simulink model "Robot"  (R2019b)
settings: Solver=VariableStepAuto  StartTime=0.0  StopTime=20  RelTol=1e-3
undefined symbols (not defined in the file or in its folder): X, Y, Z
libraries: sm_lib x11, nesl_utility x7
settings Model: Creator=Usuario  LastModifiedBy=Usuario

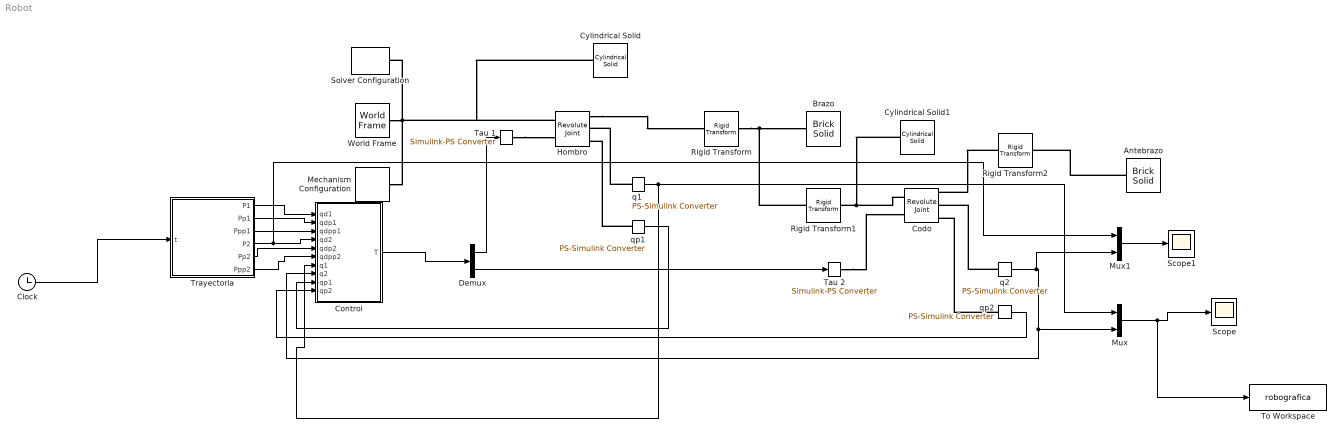
== system Robot ==
  " Brazo" : sm_lib/Body Elements/Brick Solid  GraphicAmbientColor=[0.15 0.15 0.15 1.0]  BasedOnType=Density  BrickDimensions=[0.1 1 0.1]  BrickDimensionUnits=m  CenterOfMass=[0 0 0]  CenterOfMassUnits=m  GraphicDiffuseColor=[1.0 0.2 0.2]  Density=1000  DensityUnits=kg/m^3  DoExposeReferenceFrame=on  GraphicEmissiveColor=[0.0 0.0 0.0 1.0]  ExportEntireGeometry=off  SerializedFrames=<Frames/>  MarkerShape=Sphere  MarkerSize=10  GraphicType=FromGeometry  InertiaType=Custom  Mass=1  MassUnits=kg  MomentsOfInertia=[1 1 0.01]  MomentsOfInertiaUnits=kg*m^2  GraphicOpacity=1.0  ProductsOfInertia=[0 0 0]  ProductsOfInertiaUnits=kg*m^2  GraphicShininess=75  GraphicSpecularColor=[0.5 0.5 0.5 1.0]  GraphicVisPropType=SimpleVisualProperties
  Antebrazo : sm_lib/Body Elements/Brick Solid  GraphicAmbientColor=[0.15 0.15 0.15 1.0]  BasedOnType=Density  BrickDimensions=[0.1 1 0.1]  BrickDimensionUnits=m  CenterOfMass=[0 0 0]  CenterOfMassUnits=m  GraphicDiffuseColor=[0.0 0.0 1.0]  Density=1000  DensityUnits=kg/m^3  DoExposeReferenceFrame=on  GraphicEmissiveColor=[0.0 0.0 0.0 1.0]  ExportEntireGeometry=off  SerializedFrames=<Frames/>  MarkerShape=Sphere  MarkerSize=10  GraphicType=FromGeometry  InertiaType=Custom  Mass=1  MassUnits=kg  MomentsOfInertia=[1 1 0.01]  MomentsOfInertiaUnits=kg*m^2  GraphicOpacity=1.0  ProductsOfInertia=[0 0 0]  ProductsOfInertiaUnits=kg*m^2  GraphicShininess=75  GraphicSpecularColor=[0.5 0.5 0.5 1.0]  GraphicVisPropType=SimpleVisualProperties
  Clock : Clock
  Codo : sm_lib/Joints/Revolute Joint  JointMode=Normal  SenseConstraintForce=off  SenseConstraintForceX=off  SenseConstraintForceY=off  SenseConstraintForceZ=off  SenseConstraintTorque=off  SenseConstraintTorqueX=off  SenseConstraintTorqueY=off  SenseConstraintTorqueZ=off  SenseTotalForce=off  SenseTotalForceX=off  SenseTotalForceY=off  SenseTotalForceZ=off  SenseTotalTorque=off  SenseTotalTorqueX=off  SenseTotalTorqueY=off  SenseTotalTorqueZ=off  CompositeWrenchDir=FollowerOnBase  CompositeWrenchFrame=BaseFrame  EquilibriumPosition=0  EquilibriumPositionUnits=deg  SpringStiffness=0  SpringStiffnessUnits=N*m/deg  DampingCoefficient=0.13  DampingCoefficientUnits=N*m/(rad/s)  TorqueActuationMode=InputTorque  MotionActuationMode=ComputedMotion  SensePosition=on  SenseVelocity=on  SenseAcceleration=off  SenseTorqueForce=off  SenseLowerLimitTorqueForce=off  SenseUpperLimitTorqueForce=off  LowerLimitSpecify=off  LowerLimitBound=-90  LowerLimitBoundUnits=deg  LowerLimitStiffness=1e4  LowerLimitStiffnessUnits=N*m/deg  LowerLimitDamping=10  LowerLimitDampingUnits=N*m/(deg/s)  LowerLimitTransitionRegionWidth=0.1  LowerLimitTransitionRegionWidthUnits=deg  UpperLimitSpecify=off  UpperLimitBound=90  UpperLimitBoundUnits=deg  UpperLimitStiffness=1e4  UpperLimitStiffnessUnits=N*m/deg  UpperLimitDamping=10  UpperLimitDampingUnits=N*m/(deg/s)  UpperLimitTransitionRegionWidth=0.1  UpperLimitTransitionRegionWidthUnits=deg  PositionTargetSpecify=on  PositionTargetPriority=High  PositionTargetValue=-pi/2  PositionTargetValueUnits=rad  VelocityTargetSpecify=off  VelocityTargetPriority=High  VelocityTargetValue=0  VelocityTargetValueUnits=deg/s
  Control : MATLAB Function  TreatAsAtomicUnit=on
  Cylindrical Solid : sm_lib/Body Elements/Cylindrical Solid  GraphicAmbientColor=[0.15 0.15 0.15 1.0]  BasedOnType=Density  CenterOfMass=[0 0 0]  CenterOfMassUnits=m  GraphicDiffuseColor=[1.0 1.0 0.0]  CylinderLength=0.12  CylinderLengthUnits=m  CylinderRadius=0.05  CylinderRadiusUnits=m  Density=1000  DensityUnits=kg/m^3  DoExposeReferenceFrame=on  GraphicEmissiveColor=[0.0 0.0 0.0 1.0]  ExportEntireGeometry=off  SerializedFrames=<Frames/>  MarkerShape=Sphere  MarkerSize=10  GraphicType=FromGeometry  InertiaType=Custom  Mass=0.0001  MassUnits=kg  MomentsOfInertia=[1 1 0.001]  MomentsOfInertiaUnits=kg*m^2  GraphicOpacity=1.0  ProductsOfInertia=[0 0 0]  ProductsOfInertiaUnits=kg*m^2  GraphicShininess=75  GraphicSpecularColor=[0.5 0.5 0.5 1.0]  GraphicVisPropType=SimpleVisualProperties
  Cylindrical Solid1 : sm_lib/Body Elements/Cylindrical Solid  GraphicAmbientColor=[0.15 0.15 0.15 1.0]  BasedOnType=Density  CenterOfMass=[0 0 0]  CenterOfMassUnits=m  GraphicDiffuseColor=[1.0 1.0 0.0]  CylinderLength=0.12  CylinderLengthUnits=m  CylinderRadius=0.05  CylinderRadiusUnits=m  Density=1000  DensityUnits=kg/m^3  DoExposeReferenceFrame=on  GraphicEmissiveColor=[0.0 0.0 0.0 1.0]  ExportEntireGeometry=off  SerializedFrames=<Frames/>  MarkerShape=Sphere  MarkerSize=10  GraphicType=FromGeometry  InertiaType=Custom  Mass=0.0001  MassUnits=kg  MomentsOfInertia=[1 1 0.001]  MomentsOfInertiaUnits=kg*m^2  GraphicOpacity=1.0  ProductsOfInertia=[0 0 0]  ProductsOfInertiaUnits=kg*m^2  GraphicShininess=75  GraphicSpecularColor=[0.5 0.5 0.5 1.0]  GraphicVisPropType=SimpleVisualProperties
  Demux : Demux  Outputs=2
  Hombro : sm_lib/Joints/Revolute Joint  JointMode=Normal  SenseConstraintForce=off  SenseConstraintForceX=off  SenseConstraintForceY=off  SenseConstraintForceZ=off  SenseConstraintTorque=off  SenseConstraintTorqueX=off  SenseConstraintTorqueY=off  SenseConstraintTorqueZ=off  SenseTotalForce=off  SenseTotalForceX=off  SenseTotalForceY=off  SenseTotalForceZ=off  SenseTotalTorque=off  SenseTotalTorqueX=off  SenseTotalTorqueY=off  SenseTotalTorqueZ=off  CompositeWrenchDir=FollowerOnBase  CompositeWrenchFrame=BaseFrame  EquilibriumPosition=0  EquilibriumPositionUnits=deg  SpringStiffness=0  SpringStiffnessUnits=N*m/deg  DampingCoefficient=0.17  DampingCoefficientUnits=N*m/(rad/s)  TorqueActuationMode=InputTorque  MotionActuationMode=ComputedMotion  SensePosition=on  SenseVelocity=on  SenseAcceleration=off  SenseTorqueForce=off  SenseLowerLimitTorqueForce=off  SenseUpperLimitTorqueForce=off  LowerLimitSpecify=off  LowerLimitBound=-90  LowerLimitBoundUnits=deg  LowerLimitStiffness=1e4  LowerLimitStiffnessUnits=N*m/deg  LowerLimitDamping=10  LowerLimitDampingUnits=N*m/(deg/s)  LowerLimitTransitionRegionWidth=0.1  LowerLimitTransitionRegionWidthUnits=deg  UpperLimitSpecify=off  UpperLimitBound=90  UpperLimitBoundUnits=deg  UpperLimitStiffness=1e4  UpperLimitStiffnessUnits=N*m/deg  UpperLimitDamping=10  UpperLimitDampingUnits=N*m/(deg/s)  UpperLimitTransitionRegionWidth=0.1  UpperLimitTransitionRegionWidthUnits=deg  PositionTargetSpecify=off  PositionTargetPriority=High  PositionTargetValue=pi/2  PositionTargetValueUnits=rad  VelocityTargetSpecify=off  VelocityTargetPriority=High  VelocityTargetValue=0  VelocityTargetValueUnits=deg/s
  Mechanism Configuration : sm_lib/Utilities/Mechanism Configuration  UniformGravity=Constant  GravityVector=[0 -9.80665 0]  GravityUnits=m/s^2  LinearizationDelta=0.001
  Mux : Mux  Inputs=2
  Mux1 : Mux  Inputs=2
  Rigid Transform : sm_lib/Frames and Transforms/Rigid Transform  TranslationMethod=Cartesian  TranslationStandardOffset=0  TranslationLengthUnit=m  TranslationStandardAxis=+Z  TranslationCartesianOffset=[0 -0.5 0]  TranslationROffset=0  TranslationROffsetUnits=m  TranslationZOffset=0  TranslationZOffsetUnits=m  TranslationThetaOffset=0  TranslationThetaOffsetUnits=deg  RotationMethod=None  RotationAngleUnits=deg  RotationStandardAxis=+Z  RotationAngle=0.0  RotationArbitraryAxis=[0 0 1]  FollAlignAxisA=+X  BaseAlignAxisA=+Y  FollAlignAxisB=+Y  BaseAlignAxisB=+Z  RotationSequenceAxes=FollowerAxes  RotationSequence=XYX  RotationSequenceAngles=[0 0 0]  RotationSequenceAnglesUnits=deg  RotationMatrix=[1 0 0; 0 1 0; 0 0 1]
  Rigid Transform1 : sm_lib/Frames and Transforms/Rigid Transform  TranslationMethod=Cartesian  TranslationStandardOffset=0  TranslationLengthUnit=m  TranslationStandardAxis=+Z  TranslationCartesianOffset=[0 -0.5 0]  TranslationROffset=0  TranslationROffsetUnits=m  TranslationZOffset=0  TranslationZOffsetUnits=m  TranslationThetaOffset=0  TranslationThetaOffsetUnits=deg  RotationMethod=None  RotationAngleUnits=deg  RotationStandardAxis=+Z  RotationAngle=0.0  RotationArbitraryAxis=[0 0 1]  FollAlignAxisA=+X  BaseAlignAxisA=+Y  FollAlignAxisB=+Y  BaseAlignAxisB=+Z  RotationSequenceAxes=FollowerAxes  RotationSequence=XYX  RotationSequenceAngles=[0 0 0]  RotationSequenceAnglesUnits=deg  RotationMatrix=[1 0 0; 0 1 0; 0 0 1]
  Rigid Transform2 : sm_lib/Frames and Transforms/Rigid Transform  TranslationMethod=Cartesian  TranslationStandardOffset=0  TranslationLengthUnit=m  TranslationStandardAxis=+Z  TranslationCartesianOffset=[0 -0.5 0]  TranslationROffset=0  TranslationROffsetUnits=m  TranslationZOffset=0  TranslationZOffsetUnits=m  TranslationThetaOffset=0  TranslationThetaOffsetUnits=deg  RotationMethod=None  RotationAngleUnits=deg  RotationStandardAxis=+Z  RotationAngle=0.0  RotationArbitraryAxis=[0 0 1]  FollAlignAxisA=+X  BaseAlignAxisA=+Y  FollAlignAxisB=+Y  BaseAlignAxisB=+Z  RotationSequenceAxes=FollowerAxes  RotationSequence=XYX  RotationSequenceAngles=[0 0 0]  RotationSequenceAnglesUnits=deg  RotationMatrix=[1 0 0; 0 1 0; 0 0 1]
  Scope : Scope
  Scope1 : Scope
  Solver Configuration : nesl_utility/Solver Configuration  PhysicalDomain=network_engine_domain  SubClassName=solver  LeftPortType=input  RightPortType=generic  Tones=[]  Harmonics=[]  SimulateNoise=off  Profile=off  UseLocalSampling=off  EnableSwitchedLinearOptims=on  FrequencyDomain=off  UseCCode=off  RelTol=0.001  AbsTol=1e-06  MinStep=1e-09  ToWorkspace=off  RevertToSquareIcSolve=off  NumHomotopyIterations=100  PhasorMode=off  PhasorModeNumHarmonics=1  DoDC=off  ResidualTolerance=1e-09  UseLocalSolver=off  LocalSolverChoice=NE_BACKWARD_EULER_ADVANCER  LocalSolverSampleTime=0.001  DoFixedCost=off  MaxNonlinIter=3  MaxModeIter=2  LinearAlgebra=auto  EquationFormulation=NE_TIME_EF  DelaysMemoryBudget=1024  AutomaticFiltering=on  FilteringTimeConstant=0.001  PartitionStorageMethod=AS_NEEDED  PartitionMemoryBudget=1024  PartitionMethod=ROBUST
  Tau 1 : nesl_utility/Simulink-PS Converter  PhysicalDomain=network_engine_domain  SubClassName=ps_input  LeftPortType=input  RightPortType=output  PseudoPeriodic=off  Frequencies=[]  NoiseDistribution=none  NoiseParameters=[]  Unit=N*m  AffineConversion=off  FilteringAndDerivatives=provide  SimscapeFilterOrder=1  InputFilterTimeConstant=0.001  UdotUserProvided=0
  Tau 2 : nesl_utility/Simulink-PS Converter  PhysicalDomain=network_engine_domain  SubClassName=ps_input  LeftPortType=input  RightPortType=output  PseudoPeriodic=off  Frequencies=[]  NoiseDistribution=none  NoiseParameters=[]  Unit=N*m  AffineConversion=off  FilteringAndDerivatives=provide  SimscapeFilterOrder=1  InputFilterTimeConstant=0.001  UdotUserProvided=0
  To Workspace : ToWorkspace  VariableName=robografica  SaveFormat=Timeseries  SampleTime=-1
  "Trayectoria " : MATLAB Function  TreatAsAtomicUnit=on
  World Frame : sm_lib/Frames and Transforms/World Frame
  "q1 " : nesl_utility/PS-Simulink Converter  PhysicalDomain=network_engine_domain  SubClassName=ps_output  LeftPortType=input  RightPortType=output  PseudoPeriodic=off  Frequencies=[]  Unit=rad  AffineConversion=off
  q2 : nesl_utility/PS-Simulink Converter  PhysicalDomain=network_engine_domain  SubClassName=ps_output  LeftPortType=input  RightPortType=output  PseudoPeriodic=off  Frequencies=[]  Unit=rad  AffineConversion=off
  qp1 : nesl_utility/PS-Simulink Converter  PhysicalDomain=network_engine_domain  SubClassName=ps_output  LeftPortType=input  RightPortType=output  PseudoPeriodic=off  Frequencies=[]  Unit=rad/s  AffineConversion=off
  qp2 : nesl_utility/PS-Simulink Converter  PhysicalDomain=network_engine_domain  SubClassName=ps_output  LeftPortType=input  RightPortType=output  PseudoPeriodic=off  Frequencies=[]  Unit=rad/s  AffineConversion=off
  wires:
  Mux/1 -> To Workspace/1, Scope/1
  q2/1 -> Mux1/2, Control/8(q2), Mux/2
  Demux/2 -> Tau 2/1
  Demux/1 -> Tau 1/1
  Control/1(T) -> Demux/1
  qp1/1 -> Control/9(qp1)
  qp2/1 -> Control/10(qp2)
  Clock/1 -> "Trayectoria "/1(t)
  "q1 "/1 -> Control/7(q1), Mux/1
  "Trayectoria "/1(P1) -> Control/1(qd1)
  "Trayectoria "/2(Pp1) -> Control/2(qdp1)
  "Trayectoria "/3(Ppp1) -> Control/3(qdpp1)
  "Trayectoria "/4(P2) -> Mux1/1, Control/4(qd2)
  "Trayectoria "/5(Pp2) -> Control/5(qdp2)
  "Trayectoria "/6(Ppp2) -> Control/6(qdpp2)
  Mux1/1 -> Scope1/1
  connections:
  Mechanism Configuration/RConn1 -- Cylindrical Solid/RConn1 -- Hombro/LConn1 -- World Frame/RConn1 -- Solver Configuration/RConn1
  Hombro/RConn1 -- Rigid Transform/LConn1
  Rigid Transform/RConn1 -- Rigid Transform1/LConn1 -- " Brazo"/RConn1
  Codo/LConn1 -- Cylindrical Solid1/RConn1 -- Rigid Transform1/RConn1
  Rigid Transform2/LConn1 -- Codo/RConn1
  Antebrazo/RConn1 -- Rigid Transform2/RConn1
  "q1 "/LConn1 -- Hombro/RConn2
  qp1/LConn1 -- Hombro/RConn3
  Tau 1/RConn1 -- Hombro/LConn2
  q2/LConn1 -- Codo/RConn2
  qp2/LConn1 -- Codo/RConn3
  Tau 2/RConn1 -- Codo/LConn2

== matlab function Robot/Trayectoria  ==
  data: t input; P1 output; Pp1 output; Ppp1 output; P2 output; Pp2 output; Ppp2 output
function [P1,Pp1,Ppp1,P2,Pp2,Ppp2] = fcn(t)
%Primer trayectoria

%%Parametros
teta0=0;
tetaf=pi;
teta0p=0;
tetafp=0;
teta0pp=0;
tetafpp=0;
tf=10;
%%Coeficientes
a0=teta0;
a1=teta0p;
a2=teta0pp/2;
a3=(20*tetaf-20*teta0-(8*tetafp+12*teta0p)*tf-(3*teta0pp-tetafpp)*tf^2)/(2*tf^3);
a4=(30*teta0-30*tetaf+(14*tetafp+16*teta0p)*tf+(3*teta0pp-2*tetafpp)*tf^2)/(2*tf^4);
a5=(12*tetaf-12*teta0-(6*tetafp+6*teta0p)*tf-(teta0pp-tetafpp)*tf^2)/(2*tf^5);

%%Polinomio de 5 grado
if t<=tf
P1 = a0+a1*t+a2*t^2+a3*t^3+a4*t^4+a5*t^5;
Pp1 = a1+2*a2*t+3*a3*t^2+4*a4*t^3+5*a5*t^4;
Ppp1 = 2*a2+6*a3*t+12*a4*t^2+20*a5*t^3;
else
    P1=tetaf;
    Pp1=tetafp;
    Ppp1=tetafpp;
end


%Segunda trayectoria

%%Parametros
teta0a=-pi/2;
tetafa=pi/2;
teta0p=0;
tetafp=0;
teta0pp=0;
tetafpp=0;
tfa=15;
%%Coeficientes
aa0=teta0a;
aa1=teta0p;
aa2=teta0pp/2;
aa3=(20*tetafa-20*teta0a-(8*tetafp+12*teta0p)*tfa-(3*teta0pp-tetafpp)*tfa^2)/(2*tfa^3);
aa4=(30*teta0a-30*tetafa+(14*tetafp+16*teta0p)*tfa+(3*teta0pp-2*tetafpp)*tfa^2)/(2*tfa^4);
aa5=(12*tetafa-12*teta0a-(6*tetafp+6*teta0p)*tfa-(teta0pp-tetafpp)*tfa^2)/(2*tfa^5);

%%Polinomio de 5 grado
if t<=tfa
P2 = aa0+a1*t+aa2*t^2+aa3*t^3+aa4*t^4+aa5*t^5;
Pp2 = aa1+2*aa2*t+3*aa3*t^2+4*aa4*t^3+5*aa5*t^4;
Ppp2 = 2*aa2+6*aa3*t+12*aa4*t^2+20*aa5*t^3;
else
    P2=tetafa;
    Pp2=tetafp;
    Ppp2=tetafpp;
end

== matlab function Robot/Control ==
  data: qd1 input; qdp1 input; qdpp1 input; qd2 input; qdp2 input; qdpp2 input; q1 input; T output; q2 input; qp1 input; qp2 input
function T = fcn(qd1,qdp1,qdpp1,qd2,qdp2,qdpp2,q1,q2,qp1,qp2)
% %%Parametros
% m1=1;l1=1;lc1=0.5;I1=0.01;b1=0.17;
% m2=1;l2=1;lc2=0.5;I2=0.01;b2=0.13;
% g=9.81;
% kp1=15;kp2=10;
% kd1=10;kd2=6;
% %%Ganancias
% Kp11=kp1;
% Kp12=0;
% Kp21=0;
% Kp22=kp2;
% Kp=[Kp11 Kp12;Kp21 Kp22];
% 
% Kd11=kd1;
% Kd12=0;
% Kd21=0;
% Kd22=kp2;
% Kd=[Kd11 Kd12;Kd21 Kd22];
% %%Vector de posicion
% qd1=pi;qd2=0;
% 
% qh=[qd1-q1;qd2-q2];
% qp=[qp1;qp2];
% %%Vector de gravedad
% G1=(m1*lc1+m2*l1)*g*sin(q1)+m2*g*lc2*sin(q1+q2);
% G2=m2*g*lc2*sin(q1+q2);
% G=[G1;G2];
% 
% %%Control P con retro de velocidad mas compesacion de gravedad
% T= Kp*qh-Kd*qp+G;

%%Parametros
m1=1;l1=1;lc1=0.5;I1=0.01;b1=0.17;
m2=1;l2=1;lc2=0.5;I2=0.01;b2=0.13;
g=9.81;
%%Matriz de masas
M11=m1*lc1^2+m2*l1^2+m2*lc2^2+2*m2*l1*lc2*cos(q2)+I1+I2;
M12=m2*lc2^2+m2*l1*lc2*cos(q2)+I2;
M21=m2*lc2^2+m2*l1*lc2*cos(q2)+I2;
M22=m2*lc2^2+I2;
M=[M11 M12;M21 M22];
%%Matriz de inercia
C11=-2*m2*l1*lc2*sin(q2)*qp2;
C12=-m2*l1*lc2*sin(q2)*qp2;
C21=-m2*l1*lc2*sin(q2)*qp1;
C22=0;
C = [C11 C12;C21 C22];
%%Matriz diagonal de friccion viscoza
B11=b1;
B12=0;
B21=0;
B22=b2;
B=[B11 B12;B21 B22];
%%Vector de gravedad
G1=(m1*lc1+m2*l1)*g*sin(q1)+m2*g*lc2*sin(q1+q2);
G2=m2*g*lc2*sin(q1+q2);
G=[G1;G2];

kp1=15;kp2=10;
kd1=10;kd2=6;
%%Ganancias
Kp11=kp1;
Kp12=0;
Kp21=0;
Kp22=kp2;
Kp=[Kp11 Kp12;Kp21 Kp22];

Kd11=kd1;
Kd12=0;
Kd21=0;
Kd22=kd2;
Kd=[Kd11 Kd12;Kd21 Kd22];
%%Vector de error posicion
qh=[qd1-q1;qd2-q2];
%%Vector de velocidad
qp=[qp1;qp2];
%%Vector de aceleracion deseada
qdpp=[qdpp1;qdpp2];
%%Vector del error de velocidad
qhp=[qdp1-qp1;qdp2-qp2];
%%Control de par calculado
T=M*(qdpp+Kd*qhp+Kp*qh)+C*qp+B*qp+G;
